simulink subsystem "Sun"  (R2022a)
settings: Solver=VariableStepAuto  StartTime=0.0  StopTime=10.0  RelTol=1e-3
values from neighbouring files (symbols this model uses):
  z = vec_B(3)    [SunSensor.m]    (also in backend.m = SunB.signals.values(3))
undefined symbols (not defined in the file or in its folder): sig_ss
libraries: matrix_library x2, simulink_extras x1
settings Model: Creator=emmamarsden  LastModifiedBy=emmamarsden

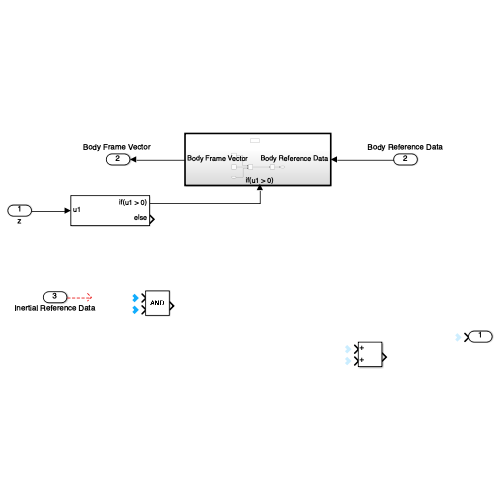
[thumbnail: Simulink's stored preview of the top-level diagram]
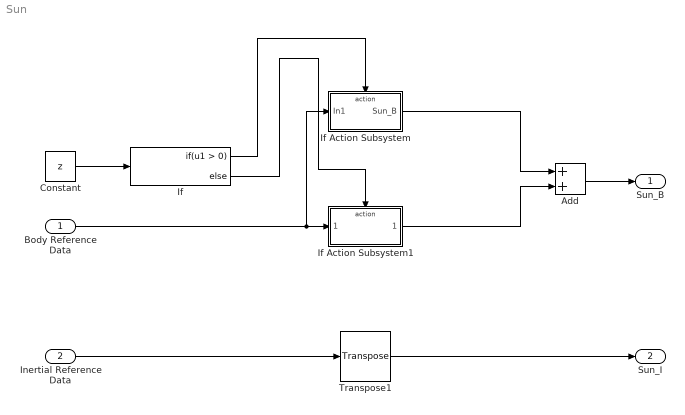
== system Sun ==
  Body Reference Data : Inport
  Inertial Reference Data : Inport  Port=2
  Add : Sum
  Constant : Constant  Value=z
  If : If
  If Action Subsystem : Subsystem  TreatAsAtomicUnit=on
  If Action Subsystem1 : Subsystem  TreatAsAtomicUnit=on
  Transpose1 : matrix_library/Transpose
      settings: SourceProductBaseCode=SL
  Sun_B : Outport
  Sun_I : Outport  Port=2
  wires:
  Inertial Reference Data/1 -> Transpose1/1
  Constant/1 -> If/1
  If/1 -> If Action Subsystem/Action
  Body Reference Data/1 -> If Action Subsystem/1(In1), If Action Subsystem1/1(Body Reference Data)
  If/2 -> If Action Subsystem1/Action
  If Action Subsystem1/1(Sun_B1) -> Add/2
  If Action Subsystem/1(Sun_B) -> Add/1
  Transpose1/1 -> Sun_I/1
  Add/1 -> Sun_B/1

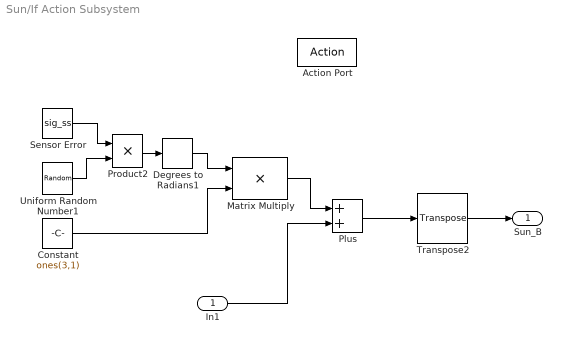
== system Sun/If Action Subsystem ==
  In1 : Inport
  Action Port : ActionPort
  Constant : Constant  Value=ones(3,1)  VectorParams1D=off
  Degrees to Radians1 : simulink_extras/Transformations/Degrees to Radians
  Matrix Multiply : Product
  Plus : Sum
  Product2 : Product
  Sensor Error : Constant  Value=sig_ss
  Transpose2 : matrix_library/Transpose
      settings: SourceProductBaseCode=SL
  Uniform Random Number1 : UniformRandomNumber  SampleTime=0.1
  Sun_B : Outport
  wires:
  Degrees to Radians1/1 -> Matrix Multiply/1
  Constant/1 -> Matrix Multiply/2
  Transpose2/1 -> Sun_B/1
  In1/1 -> Plus/2
  Product2/1 -> Degrees to Radians1/1
  Plus/1 -> Transpose2/1
  Uniform Random Number1/1 -> Product2/2
  Matrix Multiply/1 -> Plus/1
  Sensor Error/1 -> Product2/1

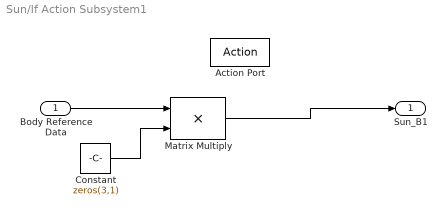
== system Sun/If Action Subsystem1 ==
  Body Reference Data : Inport
  Action Port : ActionPort
  Constant : Constant  Value=zeros(3,1)  VectorParams1D=off
  Matrix Multiply : Product
  Sun_B1 : Outport
  wires:
  Constant/1 -> Matrix Multiply/2
  Matrix Multiply/1 -> Sun_B1/1
  Body Reference Data/1 -> Matrix Multiply/1
